simulink model "trolleypitchmodel"  (R2023b)
settings: Solver=VariableStepAuto  StartTime=0.0  StopTime=10.0  RelTol=1e-3
undefined symbols (not defined in the file): csf, csr, ksf, ksr, lf, lr, mb
settings Model: Creator=ADMIN  LastModifiedBy=ADMIN

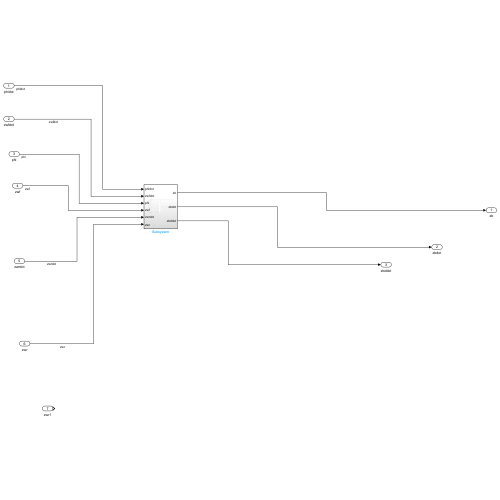
[thumbnail: Simulink's stored preview of the top-level diagram]
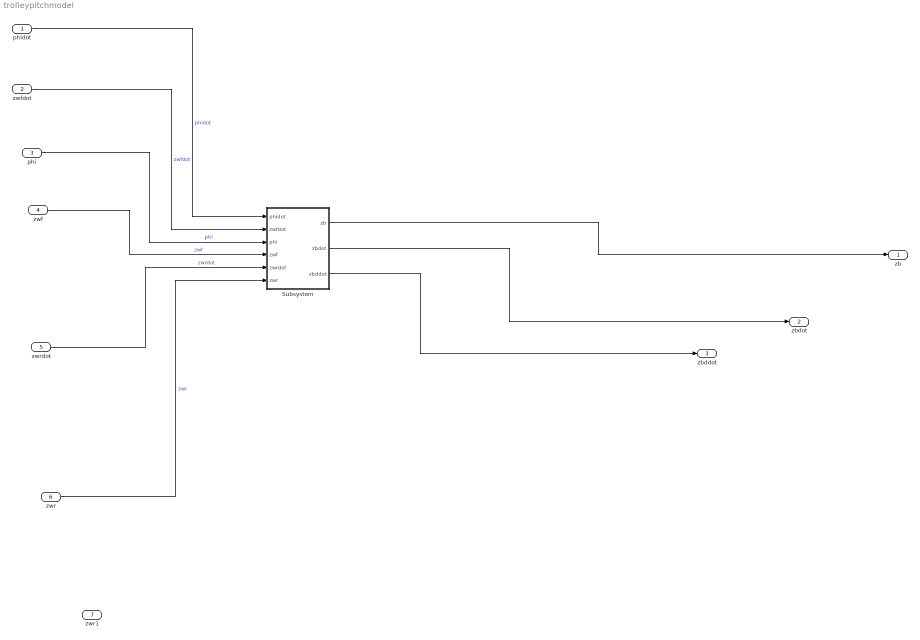
== system trolleypitchmodel ==
  phidot : Inport
  zwfdot : Inport  Port=2
  phi : Inport  Port=3
  zwf : Inport  Port=4
  zwrdot : Inport  Port=5
  zwr : Inport  Port=6
  zwr1 : Inport  Port=7
  Subsystem : Subsystem
  zb : Outport
  zbdot : Outport  Port=2
  zbddot : Outport  Port=3
  wires:
  phidot/1 -> Subsystem/1(phidot)  "phidot"
  zwfdot/1 -> Subsystem/2(zwfdot)  "zwfdot"
  phi/1 -> Subsystem/3(phi)  "phi"
  zwf/1 -> Subsystem/4(zwf)  "zwf"
  zwrdot/1 -> Subsystem/5(zwrdot)  "zwrdot"
  zwr/1 -> Subsystem/6(zwr)  "zwr"
  Subsystem/1(zb) -> zb/1
  Subsystem/2(zbdot) -> zbdot/1
  Subsystem/3(zbddot) -> zbddot/1

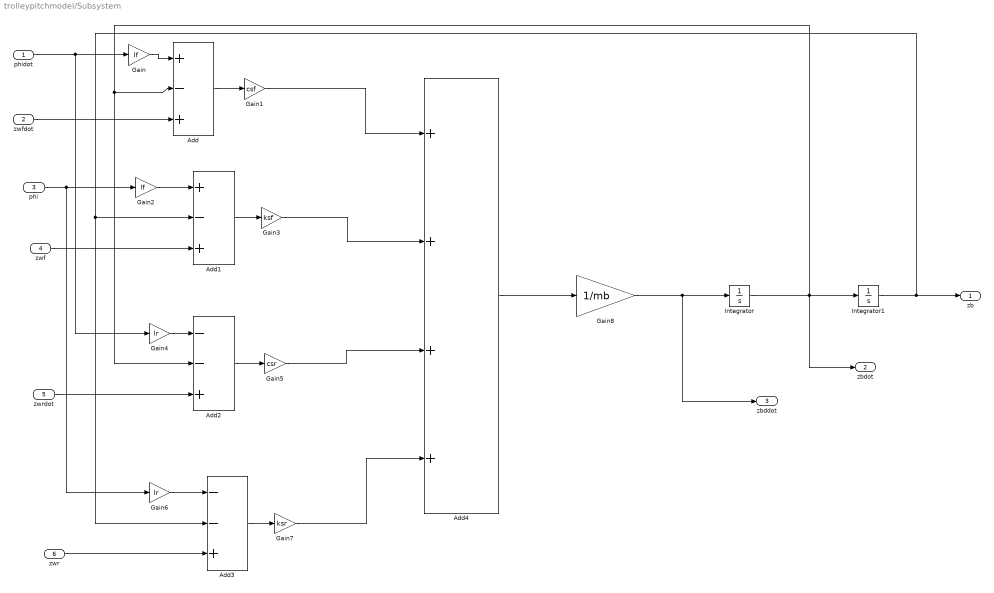
== system trolleypitchmodel/Subsystem ==
  phidot : Inport
  zwfdot : Inport  Port=2
  phi : Inport  Port=3
  zwf : Inport  Port=4
  zwrdot : Inport  Port=5
  zwr : Inport  Port=6
  Add : Sum  Inputs=+-+
  Add1 : Sum  Inputs=+-+
  Add2 : Sum  Inputs=--+
  Add3 : Sum  Inputs=--+
  Add4 : Sum  Inputs=++++
  Gain : Gain  Gain=lf
  Gain1 : Gain  Gain=csf
  Gain2 : Gain  Gain=lf
  Gain3 : Gain  Gain=ksf
  Gain4 : Gain  Gain=lr
  Gain5 : Gain  Gain=csr
  Gain6 : Gain  Gain=lr
  Gain7 : Gain  Gain=ksr
  Gain8 : Gain  Gain=1/mb
  Integrator : Integrator
  Integrator1 : Integrator
  zb : Outport
  zbdot : Outport  Port=2
  zbddot : Outport  Port=3
  wires:
  Gain/1 -> Add/1
  zwrdot/1 -> Add2/3
  Gain4/1 -> Add2/1
  phidot/1 -> Gain4/1, Gain/1
  Gain6/1 -> Add3/1
  Gain2/1 -> Add1/1
  Gain7/1 -> Add4/4
  Gain8/1 -> zbddot/1, Integrator/1
  zwfdot/1 -> Add/3
  Add/1 -> Gain1/1
  Gain3/1 -> Add4/2
  Integrator1/1 -> zb/1, Add3/2, Add1/2
  Add4/1 -> Gain8/1
  phi/1 -> Gain6/1, Gain2/1
  Add3/1 -> Gain7/1
  zwr/1 -> Add3/3
  zwf/1 -> Add1/3
  Add2/1 -> Gain5/1
  Gain1/1 -> Add4/1
  Gain5/1 -> Add4/3
  Add1/1 -> Gain3/1
  Integrator/1 -> zbdot/1, Add/2, Add2/2, Integrator1/1
